simulink model "bldc_sim_2024a_v1"  (R2024b)
settings: Solver=VariableStepAuto  StartTime=0.0  StopTime=0.5  FixedStep=1e-6  MaxStep=1e-4  RelTol=1e-3
values from neighbouring files (symbols this model uses):
  D_m = 1e-5    (= 1e-05)    [setup_motor_params.m]
  J = 12e-4    (= 0.0012)    [setup_motor_params.m]
  L_ss = 0.45e-3    (= 0.00045)    [setup_motor_params.m]
  lambda_m = 21.5e-3    (= 0.0215)    [setup_motor_params.m]
  P = 8    [setup_motor_params.m]
  phi_A_deg = 9.0 * 0    (= 0)    [setup_motor_params.m]
  phi_B_deg = -1.0 * 0    (= 0)    [setup_motor_params.m]
  phi_C_deg = 7.0* 0    (= 0)    [setup_motor_params.m]
  R_s = 0.15    [setup_motor_params.m]
  tau_s = L_ss/R_s    (= 0.003)    [setup_motor_params.m]
  Ts_motor = 1e-6    (= 1e-06)    [setup_motor_params.m]
libraries: nesl_utility x13, fl_lib x10, ee_lib x8, spsPWMGeneratorDCDCLib x2
settings Model: Creator=Aether  LastModifiedBy=Aether

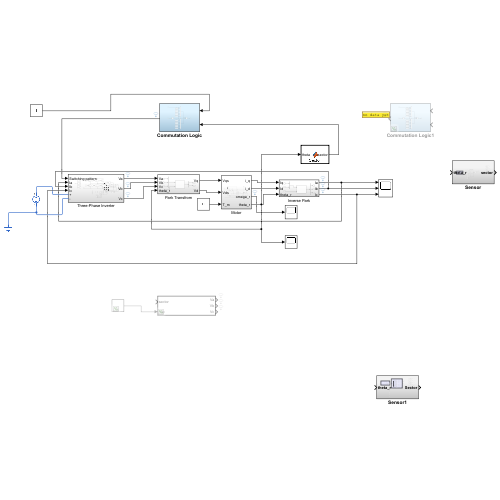
[thumbnail: Simulink's stored preview of the top-level diagram]
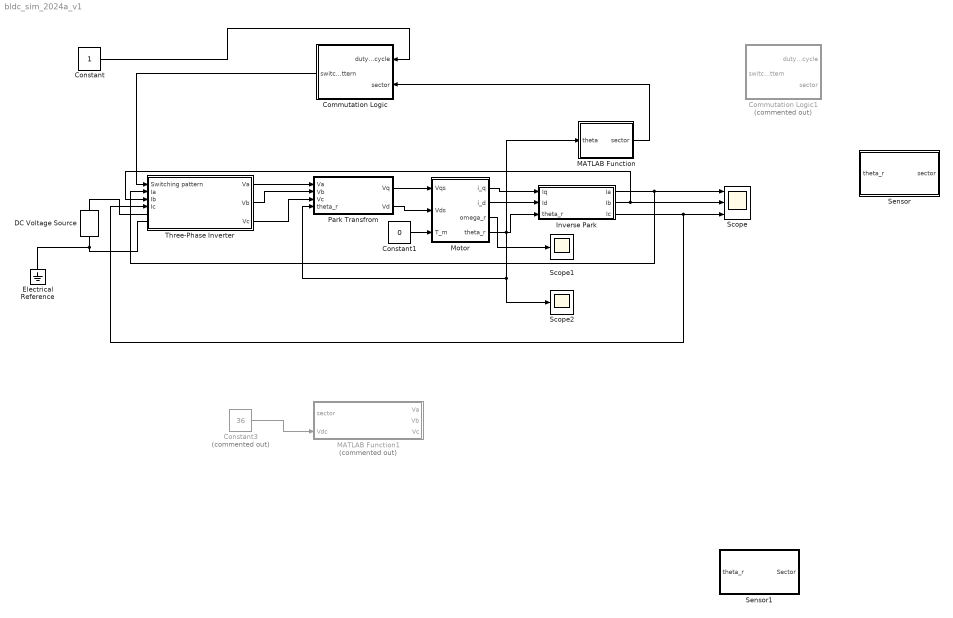
== system bldc_sim_2024a_v1 ==
  Commutation Logic : Subsystem
  Commutation Logic1 : Subsystem  Commented=on
  Constant : Constant
  Constant1 : Constant  Value=0
  Constant3 : Constant  Commented=on  Value=36
  DC Voltage Source : ee_lib/Additional Components/SPICE Sources/DC Voltage Source  DC=36 V
  Electrical Reference : fl_lib/Electrical/Electrical Elements/Electrical Reference
  Inverse Park : Subsystem
  MATLAB Function : MATLAB Function  TreatAsAtomicUnit=on
  MATLAB Function1 : MATLAB Function  Commented=on  TreatAsAtomicUnit=on
  Motor : Subsystem
  Park Transfrom : Subsystem
  Scope : Scope  NumInputPorts=3
  Scope1 : Scope
  Scope2 : Scope
  Sensor : Subsystem
  Sensor1 : Subsystem
  Three-Phase Inverter : Subsystem
  wires:
  Park Transfrom/1(Vq) -> Motor/1(Vqs)
  Park Transfrom/2(Vd) -> Motor/2(Vds)
  Motor/1(i_q) -> Inverse Park/1(Iq)
  Motor/2(i_d) -> Inverse Park/2(Id)
  Motor/4(theta_r) -> MATLAB Function/1(theta), Scope2/1, Park Transfrom/4(theta_r), Inverse Park/3(theta_r)
  Inverse Park/1(Ia) -> Three-Phase Inverter/2(Ia), Scope/1
  Inverse Park/2(Ib) -> Scope/2, Three-Phase Inverter/3(Ib)
  Inverse Park/3(Ic) -> Three-Phase Inverter/4(Ic), Scope/3
  Constant1/1 -> Motor/3(T_m)
  Motor/3(omega_r) -> Scope1/1
  Constant3/1 -> MATLAB Function1/2(Vdc)
  Three-Phase Inverter/1(Va) -> Park Transfrom/1(Va)
  Three-Phase Inverter/2(Vb) -> Park Transfrom/2(Vb)
  Three-Phase Inverter/3(Vc) -> Park Transfrom/3(Vc)
  Constant/1 -> Commutation Logic/1(duty_cycle)
  MATLAB Function/1(sector) -> Commutation Logic/2(sector)
  Commutation Logic/1("  switching_pattern") -> Three-Phase Inverter/1(Switching pattern)
  connections:
  DC Voltage Source/LConn1 -- Three-Phase Inverter/LConn1
  DC Voltage Source/RConn1 -- Electrical Reference/LConn1 -- Three-Phase Inverter/LConn2

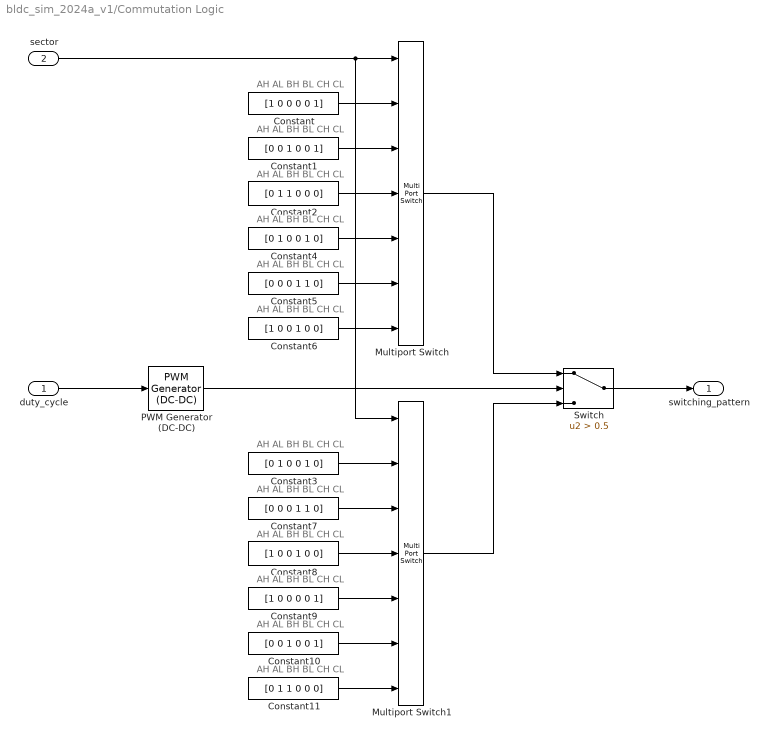
== system bldc_sim_2024a_v1/Commutation Logic ==
  note: AH AL BH BL CH CL
  note: AH AL BH BL CH CL
  note: AH AL BH BL CH CL
  note: AH AL BH BL CH CL
  note: AH AL BH BL CH CL
  note: AH AL BH BL CH CL
  note: AH AL BH BL CH CL
  note: AH AL BH BL CH CL
  note: AH AL BH BL CH CL
  note: AH AL BH BL CH CL
  note: AH AL BH BL CH CL
  note: AH AL BH BL CH CL
  duty_cycle : Inport
  sector : Inport  Port=2
  Constant : Constant  Value=[1 0 0 0 0 1]
  Constant1 : Constant  Value=[0 0 1 0 0 1]
  Constant10 : Constant  Value=[0 0 1 0 0 1]
  Constant11 : Constant  Value=[0 1 1 0 0 0]
  Constant2 : Constant  Value=[0 1 1 0 0 0]
  Constant3 : Constant  Value=[0 1 0 0 1 0]
  Constant4 : Constant  Value=[0 1 0 0 1 0]
  Constant5 : Constant  Value=[0 0 0 1 1 0]
  Constant6 : Constant  Value=[1 0 0 1 0 0]
  Constant7 : Constant  Value=[0 0 0 1 1 0]
  Constant8 : Constant  Value=[1 0 0 1 0 0]
  Constant9 : Constant  Value=[1 0 0 0 0 1]
  Multiport Switch : MultiPortSwitch  Inputs=6  SaturateOnIntegerOverflow=off  InputSameDT=off
  Multiport Switch1 : MultiPortSwitch  Inputs=6  SaturateOnIntegerOverflow=off  InputSameDT=off
  PWM Generator (DC-DC) : spsPWMGeneratorDCDCLib/PWM Generator (DC-DC)  Fsw=1e4  Ts=Ts_motor
  Switch : Switch  Criteria=u2 > Threshold  Threshold=0.5  SaturateOnIntegerOverflow=off  InputSameDT=off
  "  switching_pattern" : Outport  VectorParamsAs1DForOutWhenUnconnected=off
  wires:
  Constant6/1 -> Multiport Switch/7
  Constant4/1 -> Multiport Switch/5
  sector/1 -> Multiport Switch1/1, Multiport Switch/1
  Constant1/1 -> Multiport Switch/3
  Constant2/1 -> Multiport Switch/4
  Constant5/1 -> Multiport Switch/6
  Constant/1 -> Multiport Switch/2
  Constant9/1 -> Multiport Switch1/5
  Constant11/1 -> Multiport Switch1/7
  Constant3/1 -> Multiport Switch1/2
  Constant7/1 -> Multiport Switch1/3
  Constant10/1 -> Multiport Switch1/6
  Constant8/1 -> Multiport Switch1/4
  PWM Generator (DC-DC)/1 -> Switch/2
  Switch/1 -> "  switching_pattern"/1
  Multiport Switch/1 -> Switch/1
  Multiport Switch1/1 -> Switch/3
  duty_cycle/1 -> PWM Generator (DC-DC)/1

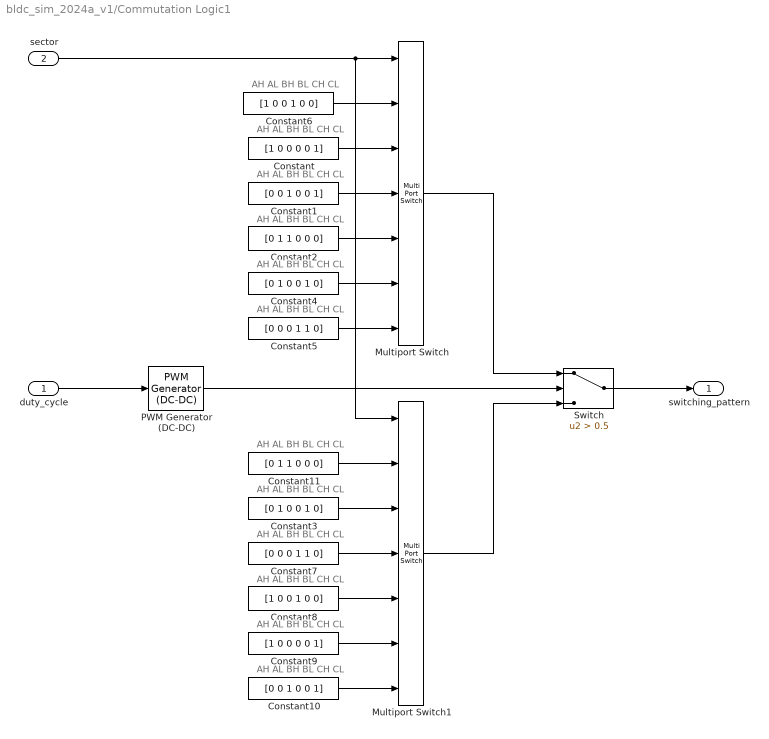
== system bldc_sim_2024a_v1/Commutation Logic1 ==
  note: AH AL BH BL CH CL
  note: AH AL BH BL CH CL
  note: AH AL BH BL CH CL
  note: AH AL BH BL CH CL
  note: AH AL BH BL CH CL
  note: AH AL BH BL CH CL
  note: AH AL BH BL CH CL
  note: AH AL BH BL CH CL
  note: AH AL BH BL CH CL
  note: AH AL BH BL CH CL
  note: AH AL BH BL CH CL
  note: AH AL BH BL CH CL
  duty_cycle : Inport
  sector : Inport  Port=2
  Constant : Constant  Value=[1 0 0 0 0 1]
  Constant1 : Constant  Value=[0 0 1 0 0 1]
  Constant10 : Constant  Value=[0 0 1 0 0 1]
  Constant11 : Constant  Value=[0 1 1 0 0 0]
  Constant2 : Constant  Value=[0 1 1 0 0 0]
  Constant3 : Constant  Value=[0 1 0 0 1 0]
  Constant4 : Constant  Value=[0 1 0 0 1 0]
  Constant5 : Constant  Value=[0 0 0 1 1 0]
  Constant6 : Constant  Value=[1 0 0 1 0 0]
  Constant7 : Constant  Value=[0 0 0 1 1 0]
  Constant8 : Constant  Value=[1 0 0 1 0 0]
  Constant9 : Constant  Value=[1 0 0 0 0 1]
  Multiport Switch : MultiPortSwitch  Inputs=6  SaturateOnIntegerOverflow=off  InputSameDT=off
  Multiport Switch1 : MultiPortSwitch  Inputs=6  SaturateOnIntegerOverflow=off  InputSameDT=off
  PWM Generator (DC-DC) : spsPWMGeneratorDCDCLib/PWM Generator (DC-DC)  Fsw=1e4  Ts=Ts_motor
  Switch : Switch  Criteria=u2 > Threshold  Threshold=0.5  SaturateOnIntegerOverflow=off  InputSameDT=off
  "  switching_pattern" : Outport  VectorParamsAs1DForOutWhenUnconnected=off
  wires:
  sector/1 -> Multiport Switch1/1, Multiport Switch/1
  PWM Generator (DC-DC)/1 -> Switch/2
  Switch/1 -> "  switching_pattern"/1
  Multiport Switch/1 -> Switch/1
  Multiport Switch1/1 -> Switch/3
  duty_cycle/1 -> PWM Generator (DC-DC)/1
  Constant5/1 -> Multiport Switch/7
  Constant4/1 -> Multiport Switch/6
  Constant2/1 -> Multiport Switch/5
  Constant1/1 -> Multiport Switch/4
  Constant/1 -> Multiport Switch/3
  Constant6/1 -> Multiport Switch/2
  Constant10/1 -> Multiport Switch1/7
  Constant9/1 -> Multiport Switch1/6
  Constant8/1 -> Multiport Switch1/5
  Constant7/1 -> Multiport Switch1/4
  Constant3/1 -> Multiport Switch1/3
  Constant11/1 -> Multiport Switch1/2

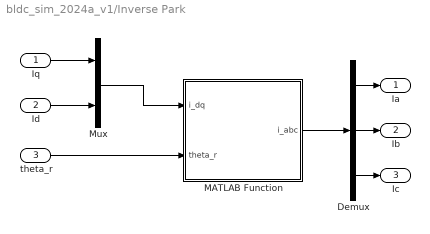
== system bldc_sim_2024a_v1/Inverse Park ==
  Iq : Inport
  Id : Inport  Port=2
  theta_r : Inport  Port=3
  Demux : Demux  Outputs=3
  MATLAB Function : MATLAB Function  TreatAsAtomicUnit=on
  Mux : Mux  Inputs=2
  Ia : Outport
  Ib : Outport  Port=2
  Ic : Outport  Port=3
  wires:
  Mux/1 -> MATLAB Function/1(i_dq)
  theta_r/1 -> MATLAB Function/2(theta_r)
  MATLAB Function/1(i_abc) -> Demux/1
  Id/1 -> Mux/2
  Iq/1 -> Mux/1
  Demux/1 -> Ia/1
  Demux/2 -> Ib/1
  Demux/3 -> Ic/1

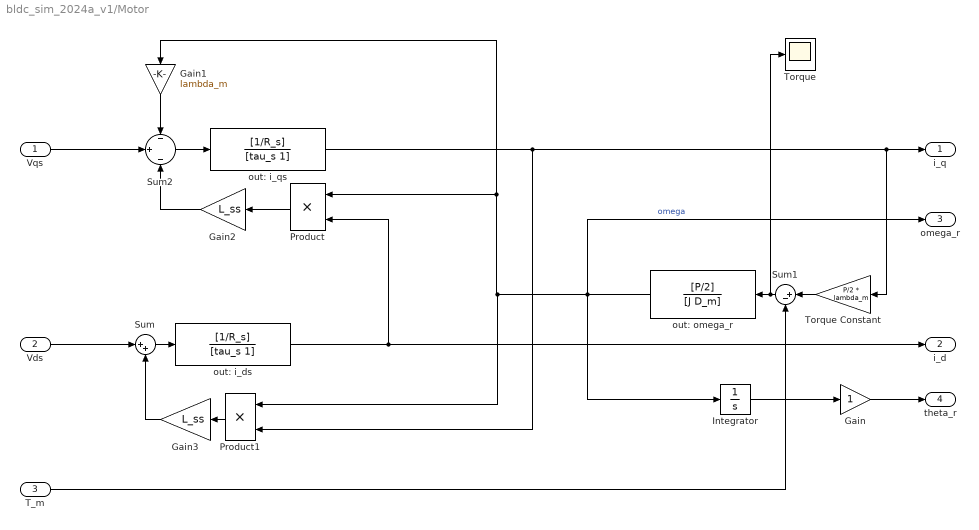
== system bldc_sim_2024a_v1/Motor ==
  Vqs : Inport
  Vds : Inport  Port=2
  T_m : Inport  Port=3
  Gain : Gain
  Gain1 : Gain  Gain=lambda_m
  Gain2 : Gain  Gain=L_ss
  Gain3 : Gain  Gain=L_ss
  Integrator : Integrator
  Product : Product
  Product1 : Product
  Sum : Sum  Inputs=|++
  Sum1 : Sum  Inputs=|+-
  Sum2 : Sum  Inputs=-|+|-
  Torque : Scope
  Torque Constant : Gain  Gain=P/2 * lambda_m
  out: i_ds : TransferFcn  Numerator=[1/R_s]  Denominator=[tau_s 1]
  out: i_qs : TransferFcn  Numerator=[1/R_s]  Denominator=[tau_s 1]
  out: omega_r : TransferFcn  Numerator=[P/2]  Denominator=[J D_m]
  i_q : Outport
  i_d : Outport  Port=2
  omega_r : Outport  Port=3
  theta_r : Outport  Port=4
  wires:
  Sum2/1 -> out: i_qs/1
  Vqs/1 -> Sum2/2
  out: omega_r/1 -> omega_r/1, Integrator/1, Product1/1, Product/1, Gain1/1  "omega"
  Gain1/1 -> Sum2/1
  out: i_ds/1 -> Product/2, i_d/1
  Integrator/1 -> Gain/1
  T_m/1 -> Sum1/2
  Sum1/1 -> Torque/1, out: omega_r/1
  Sum/1 -> out: i_ds/1
  Torque Constant/1 -> Sum1/1
  Product/1 -> Gain2/1
  out: i_qs/1 -> Product1/2, i_q/1, Torque Constant/1
  Vds/1 -> Sum/1
  Gain/1 -> theta_r/1
  Product1/1 -> Gain3/1
  Gain3/1 -> Sum/2
  Gain2/1 -> Sum2/3

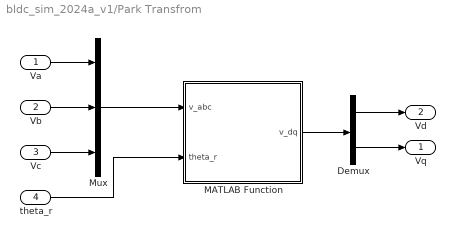
== system bldc_sim_2024a_v1/Park Transfrom ==
  Va : Inport
  Vb : Inport  Port=2
  Vc : Inport  Port=3
  theta_r : Inport  Port=4
  Demux : Demux  Outputs=2
  MATLAB Function : MATLAB Function  TreatAsAtomicUnit=on
  Mux : Mux  Inputs=3
  Vq : Outport
  Vd : Outport  Port=2
  wires:
  theta_r/1 -> MATLAB Function/2(theta_r)
  Vb/1 -> Mux/2
  Va/1 -> Mux/1
  Vc/1 -> Mux/3
  Mux/1 -> MATLAB Function/1(v_abc)
  MATLAB Function/1(v_dq) -> Demux/1
  Demux/1 -> Vd/1
  Demux/2 -> Vq/1

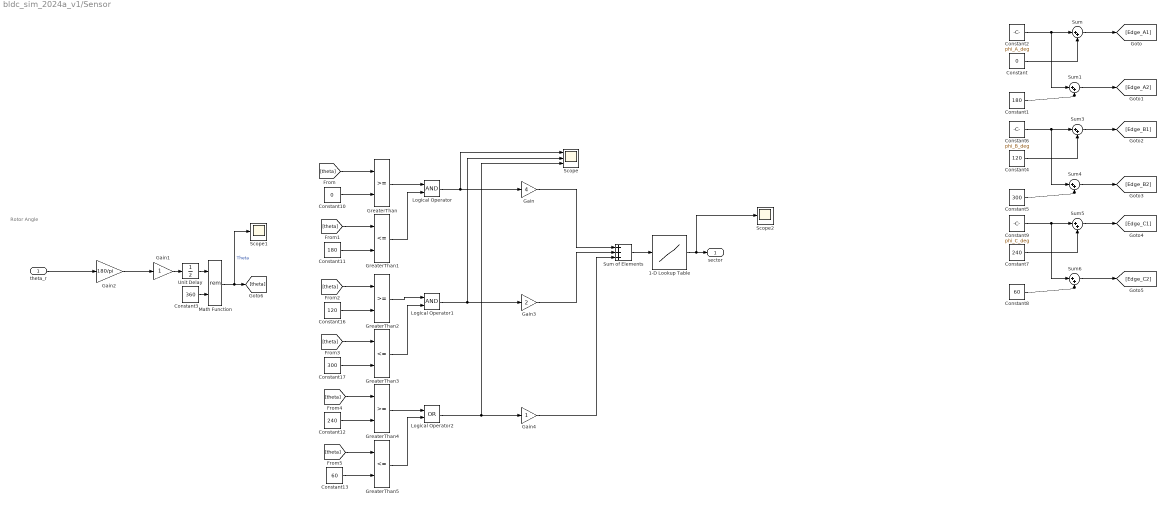
== system bldc_sim_2024a_v1/Sensor ==
  note: Rotor Angle
  theta_r : Inport
  1-D Lookup Table : Lookup_n-D  NumberOfTableDimensions=1  BreakpointsForDimension1=[1 2 3 4 5 6]  Table=[6 4 5 2 1 3]  ExtrapMethod=Clip  InternalRulePriority=Speed  RndMeth=Simplest
  Constant : Constant  Value=0
  Constant1 : Constant  Value=180
  Constant10 : Constant  Value=0
  Constant11 : Constant  Value=180
  Constant12 : Constant  Value=240
  Constant13 : Constant  Value=60
  Constant16 : Constant  Value=120
  Constant17 : Constant  Value=300
  Constant2 : Constant  Value=phi_A_deg
  Constant3 : Constant  Value=360
  Constant4 : Constant  Value=120
  Constant5 : Constant  Value=300
  Constant6 : Constant  Value=phi_B_deg
  Constant7 : Constant  Value=240
  Constant8 : Constant  Value=60
  Constant9 : Constant  Value=phi_C_deg
  Gain : Gain  Gain=4
  Gain1 : Gain
  Gain2 : Gain  Gain=180/pi
  Gain3 : Gain  Gain=2
  Gain4 : Gain
  GreaterThan : RelationalOperator  OutDataTypeStr=boolean  RndMeth=Simplest  InputSameDT=off
  GreaterThan1 : RelationalOperator  Operator=<=  OutDataTypeStr=boolean  RndMeth=Simplest  InputSameDT=off
  GreaterThan2 : RelationalOperator  OutDataTypeStr=boolean  RndMeth=Simplest  InputSameDT=off
  GreaterThan3 : RelationalOperator  Operator=<=  OutDataTypeStr=boolean  RndMeth=Simplest  InputSameDT=off
  GreaterThan4 : RelationalOperator  OutDataTypeStr=boolean  RndMeth=Simplest  InputSameDT=off
  GreaterThan5 : RelationalOperator  Operator=<=  OutDataTypeStr=boolean  RndMeth=Simplest  InputSameDT=off
  Logical Operator : Logic  AllPortsSameDT=off  OutDataTypeStr=boolean
  Logical Operator1 : Logic  AllPortsSameDT=off  OutDataTypeStr=boolean
  Logical Operator2 : Logic  Operator=OR  AllPortsSameDT=off  OutDataTypeStr=boolean
  Math Function : Math  Operator=rem  SignedPower=on
  Scope : Scope  NumInputPorts=3
  Scope1 : Scope
  Scope2 : Scope
  Sum{,1,3..6} (6 alike) : Sum  Inputs=|++
  Sum of Elements : Sum  Inputs=+++
  Unit Delay : UnitDelay  SampleTime=Ts_motor  HasFrameUpgradeWarning=on
  sector : Outport
  wires:
  Gain2/1 -> Gain1/1
  Constant3/1 -> Math Function/2
  Gain1/1 -> Unit Delay/1
  Unit Delay/1 -> Math Function/1
  Constant/1 -> Sum/2
  Constant2/1 -> Sum1/1, Sum/1
  Constant1/1 -> Sum1/2
  Sum/1 -> [Edge_A1]
  Sum1/1 -> [Edge_A2]
  Constant6/1 -> Sum4/1, Sum3/1
  Constant5/1 -> Sum4/2
  Constant4/1 -> Sum3/2
  Sum3/1 -> [Edge_B1]
  Sum4/1 -> [Edge_B2]
  Constant9/1 -> Sum6/1, Sum5/1
  Constant8/1 -> Sum6/2
  Constant7/1 -> Sum5/2
  Sum5/1 -> [Edge_C1]
  Sum6/1 -> [Edge_C2]
  theta_r/1 -> Gain2/1
  Math Function/1 -> Scope1/1, [theta]  "Theta"
  GreaterThan/1 -> Logical Operator/1
  [theta] -> GreaterThan/1
  Constant11/1 -> GreaterThan1/2
  GreaterThan1/1 -> Logical Operator/2
  GreaterThan3/1 -> Logical Operator1/2
  GreaterThan2/1 -> Logical Operator1/1
  GreaterThan4/1 -> Logical Operator2/1
  GreaterThan5/1 -> Logical Operator2/2
  Logical Operator/1 -> Scope/1, Gain/1
  Logical Operator1/1 -> Scope/2, Gain3/1
  Logical Operator2/1 -> Scope/3, Gain4/1
  Sum of Elements/1 -> 1-D Lookup Table/1
  Gain/1 -> Sum of Elements/1
  Gain3/1 -> Sum of Elements/2
  Gain4/1 -> Sum of Elements/3
  1-D Lookup Table/1 -> Scope2/1, sector/1
  Constant10/1 -> GreaterThan/2
  [theta] -> GreaterThan1/1
  [theta] -> GreaterThan2/1
  Constant16/1 -> GreaterThan2/2
  [theta] -> GreaterThan3/1
  Constant17/1 -> GreaterThan3/2
  [theta] -> GreaterThan4/1
  Constant12/1 -> GreaterThan4/2
  [theta] -> GreaterThan5/1
  Constant13/1 -> GreaterThan5/2

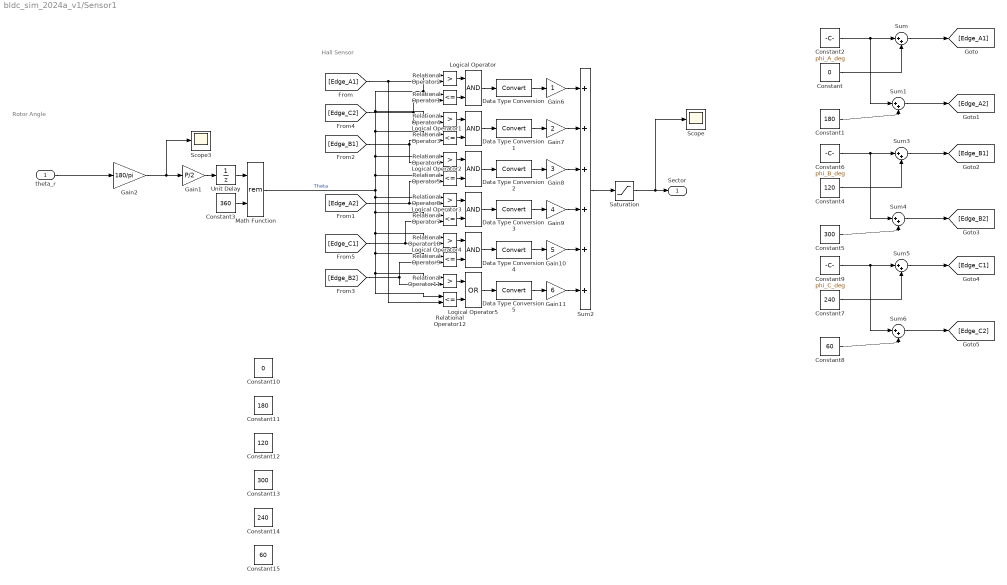
== system bldc_sim_2024a_v1/Sensor1 ==
  note: Rotor Angle
  note: Hall Sensor
  theta_r : Inport
  Constant : Constant  Value=0
  Constant1 : Constant  Value=180
  Constant10 : Constant  Value=0
  Constant11 : Constant  Value=180
  Constant12 : Constant  Value=120
  Constant13 : Constant  Value=300
  Constant14 : Constant  Value=240
  Constant15 : Constant  Value=60
  Constant2 : Constant  Value=phi_A_deg
  Constant3 : Constant  Value=360
  Constant4 : Constant  Value=120
  Constant5 : Constant  Value=300
  Constant6 : Constant  Value=phi_B_deg
  Constant7 : Constant  Value=240
  Constant8 : Constant  Value=60
  Constant9 : Constant  Value=phi_C_deg
  Data Type Conversion{,1..5} (6 alike) : DataTypeConversion
  Gain1 : Gain  Gain=P/2
  Gain10 : Gain  Gain=5  SaturateOnIntegerOverflow=on  OutDataTypeStr=Inherit: Same as input  ParamDataTypeStr=Inherit: Same as input
  Gain11 : Gain  Gain=6  SaturateOnIntegerOverflow=on  OutDataTypeStr=Inherit: Same as input  ParamDataTypeStr=Inherit: Same as input
  Gain2 : Gain  Gain=180/pi
  Gain6 : Gain  SaturateOnIntegerOverflow=on  OutDataTypeStr=Inherit: Same as input  ParamDataTypeStr=Inherit: Same as input
  Gain7 : Gain  Gain=2  SaturateOnIntegerOverflow=on  OutDataTypeStr=Inherit: Same as input  ParamDataTypeStr=Inherit: Same as input
  Gain8 : Gain  Gain=3  SaturateOnIntegerOverflow=on  OutDataTypeStr=Inherit: Same as input  ParamDataTypeStr=Inherit: Same as input
  Gain9 : Gain  Gain=4  SaturateOnIntegerOverflow=on  OutDataTypeStr=Inherit: Same as input  ParamDataTypeStr=Inherit: Same as input
  Logical Operator{,1..4} (5 alike) : Logic
  Logical Operator5 : Logic  Operator=OR
  Math Function : Math  Operator=rem  SignedPower=on
  Relational Operator{1,3,5,7,9,12} (6 alike) : RelationalOperator  Operator=<=
  Relational Operator{2,4,6,8,10..11} (6 alike) : RelationalOperator  Operator=>
  Saturation : Saturate  UpperLimit=6  LowerLimit=1
  Scope : Scope
  Scope3 : Scope
  Sum{,1,3..6} (6 alike) : Sum  Inputs=|++
  Sum2 : Sum  Inputs=++++++  InputSameDT=on  SaturateOnIntegerOverflow=on  OutDataTypeStr=Inherit: Same as first input
  Unit Delay : UnitDelay  SampleTime=Ts_motor  HasFrameUpgradeWarning=on
  Sector : Outport
  wires:
  Saturation/1 -> Scope/1, Sector/1
  Math Function/1 -> Relational Operator2/1, Relational Operator1/1, Relational Operator4/1, Relational Operator3/1, Relational Operator6/1, Relational Operator5/1, Relational Operator12/1, Relational Operator11/1, Relational Operator9/1, Relational Operator10/1, Relational Operator7/1, Relational Operator8/1  "Theta"
  Data Type Conversion5/1 -> Gain11/1
  Data Type Conversion4/1 -> Gain10/1
  Data Type Conversion3/1 -> Gain9/1
  Data Type Conversion2/1 -> Gain8/1
  Data Type Conversion1/1 -> Gain7/1
  Data Type Conversion/1 -> Gain6/1
  Relational Operator2/1 -> Logical Operator/1
  Relational Operator1/1 -> Logical Operator/2
  Logical Operator/1 -> Data Type Conversion/1
  [Edge_A1] -> Relational Operator12/2, Relational Operator2/2
  Relational Operator4/1 -> Logical Operator1/1
  Relational Operator3/1 -> Logical Operator1/2
  Logical Operator1/1 -> Data Type Conversion1/1
  [Edge_C2] -> Relational Operator1/2, Relational Operator4/2
  Relational Operator6/1 -> Logical Operator2/1
  Relational Operator5/1 -> Logical Operator2/2
  Logical Operator2/1 -> Data Type Conversion2/1
  Relational Operator8/1 -> Logical Operator3/1
  Relational Operator7/1 -> Logical Operator3/2
  Logical Operator3/1 -> Data Type Conversion3/1
  Relational Operator10/1 -> Logical Operator4/1
  Relational Operator9/1 -> Logical Operator4/2
  Logical Operator4/1 -> Data Type Conversion4/1
  Relational Operator11/1 -> Logical Operator5/1
  Relational Operator12/1 -> Logical Operator5/2
  Logical Operator5/1 -> Data Type Conversion5/1
  Gain6/1 -> Sum2/1
  Gain7/1 -> Sum2/2
  Gain8/1 -> Sum2/3
  Gain9/1 -> Sum2/4
  Gain10/1 -> Sum2/5
  Gain11/1 -> Sum2/6
  Sum2/1 -> Saturation/1
  Gain2/1 -> Scope3/1, Gain1/1
  Constant3/1 -> Math Function/2
  Gain1/1 -> Unit Delay/1
  Unit Delay/1 -> Math Function/1
  Constant/1 -> Sum/2
  Constant2/1 -> Sum1/1, Sum/1
  Constant1/1 -> Sum1/2
  Sum/1 -> [Edge_A1]
  Sum1/1 -> [Edge_A2]
  Constant6/1 -> Sum4/1, Sum3/1
  Constant5/1 -> Sum4/2
  Constant4/1 -> Sum3/2
  Sum3/1 -> [Edge_B1]
  Sum4/1 -> [Edge_B2]
  Constant9/1 -> Sum6/1, Sum5/1
  Constant8/1 -> Sum6/2
  Constant7/1 -> Sum5/2
  Sum5/1 -> [Edge_C1]
  Sum6/1 -> [Edge_C2]
  [Edge_B1] -> Relational Operator3/2, Relational Operator6/2
  [Edge_A2] -> Relational Operator5/2, Relational Operator8/2
  [Edge_C1] -> Relational Operator7/2, Relational Operator10/2
  [Edge_B2] -> Relational Operator11/2, Relational Operator9/2
  theta_r/1 -> Gain2/1

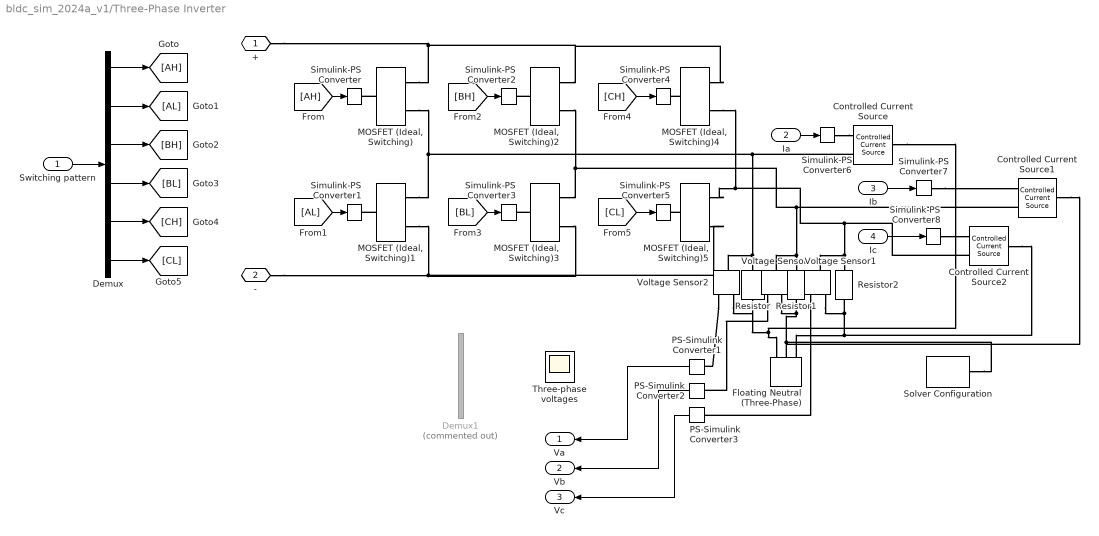
== system bldc_sim_2024a_v1/Three-Phase Inverter ==
  Switching pattern : Inport
  Ia : Inport  Port=2
  Ib : Inport  Port=3
  Ic : Inport  Port=4
  Controlled Current Source : fl_lib/Electrical/Electrical Sources/Controlled Current Source
  Controlled Current Source1 : fl_lib/Electrical/Electrical Sources/Controlled Current Source
  Controlled Current Source2 : fl_lib/Electrical/Electrical Sources/Controlled Current Source
  Demux : Demux  Outputs=6
  Demux1 : Demux  Commented=on  Outputs=3
  Floating Neutral (Three-Phase) : ee_lib/Connectors & References/Floating Neutral (Three-Phase)  G_parasitic=1e-12 1/Ohm
      settings: InternalSimscapePortConfiguration="{\"Bottom\":[],\"Left\":[{\"id\":\"a\",\"label\":\"a\",\"type\":\"foundation.electrical.electrical\"},{\"id\":\"b\",\"label\":\"b\",\"type\":\"foundation.electrical.electrical\"},{\"id\":\"c\",\"label\":\"c\",\"type\":\"foundation.electrical.electrical\"}],\"Right\":[],\"Top\":[]}"
  MOSFET (Ideal, Switching){,1..5} (6 alike) : ee_lib/Semiconductors & Converters/MOSFET (Ideal, Switching)  port_option=ee.enum.controlport.ps  Rds=0.01 Ohm  Goff=1e-6 1/Ohm  Vth=0.5 V  diode_param=ee.enum.semiconductors.protectionDiode.nodynamics  diode_Vf=0.1 V  diode_Ron=0.001 Ohm  diode_Goff=1e-5 1/Ohm  diode_C=50e-9 F  diode_iRM=-235 A  diode_iF=300 A  diode_idot=-50 A/us  diode_trr_param=ee.enum.converters.diodeReverseParam.trr_factor  diode_trr_factor=3  diode_trr=15 us  diode_Qrr=1500 s*uA  ids_specify=off  ids_priority=None  ids=0 A  ids_nominal_specify=off  ids_nominal_value=1  ids_nominal_unit=A  vds_specify=off  vds_priority=None  vds=0 V  vds_nominal_specify=off  vds_nominal_value=1  vds_nominal_unit=V  vgs_specify=off  vgs_priority=None  vgs=0 V  vgs_nominal_specify=off  vgs_nominal_value=1  vgs_nominal_unit=V  thermal_loss_option=ee.enum.converters.thermalLossOption.constantvalues  Von_data=[0, 1.8, 3.2, 6, 10, 16; 0, 2, 5.5, 9.5, 15, 25] V  Tj=[298.15, 448.15] K  Iout_data=[0, 20, 40, 60, 80, 100] A  Eon_data=[0, 55.04, 124.57, 235.53, 362.12; 0, 71.25, 161.25, 304.88, 468.75] * 1e-6 J  Eoff_data=[0, 18, 30, 56.1, 76.5; 0, 22.5, 37.5, 70.13, 95.63] * 1e-6 J  Eon_data_3D=[zeros(2, 5, 3)] J  Eoff_data_3D=[zeros(2, 5, 3)] J  Tj_loss=[298.15, 448.15] K  Iout_data_loss=[0, 10, 20, 30, 40] A  tabulateWithVds=false  Vds_loss=[0, 150, 300] V  Eon_scalar=22.86e-3 J  Eoff_scalar=17.14e-3 J  Voff=300 V  Iout_scalar=600 A  useCurrentFromPreviousCycle=false  useVoltageFromPreviousCycle=false  diodeModelType=ee.enum.converters.diodeModelType.pwl  diodeTableType=ee.enum.diode.tableType.IfMat  diode_ReverseIVType=ee.enum.diode.diodeReverseIV.constant  diode_IfMat=[.07, .12, .19, 1.75, 4.24, 7.32, 11.2; .16, .3, .72, 2.14, 4.02, 6.35, 9.12] A  diode_VfMat=[.9, 1.15, 1.25, 1.5, 1.75, 2.17, 2.6, 2.85; .58, .68, .75, 1.1, 1.38, 1.77, 2.27, 2.7] V  diode_TjVec=[25, 125] degC  diode_VfVec=[.5, .7, .9, 1.3, 1.7, 2.1, 2.5] V  diode_IfVec=[.1, .2, .5, 1, 2, 4, 7, 10] A  diode_IrMat=[1e-06, 2e-06, 5e-06, 1e-05, 2.5e-05, 5e-05, .0001; 2e-06, 5e-06, 1e-05, 4e-05, 8e-05, .0002, .0005] A  diode_VrMat=[10, 100, 200, 250, 300, 325, 350; 10, 70, 160, 220, 270, 300, 320] V  diode_VrVec=[10, 20, 40, 50, 70, 80, 100] V  diode_IrVec=[1e-06, 2e-06, 5e-06, 1e-05, 2e-05, 5e-05, .0001] A  diode_Vr=-600 V  diode_Ls=150 nH  diode_Erec=0.03 J  diode_rec_loss_model=ee.enum.diode.reverseRecoveryModel.fixed  diode_ErecVal=0 J  diode_scaleWithIandV=true  diode_ErecMat=zeros(2, 3) J  diode_TjrecVec=[298.15, 398.15] K  diode_IfrecVec=[.1, 1, 10] A  diode_IrecVal=10 A  diode_VrecVal=10 V  diode_tFilter=1 / 1000 / 100 s  separateThermalPortForDiode=false  thermal_network_parameterization=ee.enum.thermalNetworkTopology.external  Rth=[.03, .2] K/W  Rth_Cauer=[.03, .1, .2] K/W  Rth_Foster=[.03, .2] K/W  thermal_mass_parameterization=ee.enum.thermalNetwork.timeconstant  thermal_mass=[3, 25] J/K  thermal_mass_Cauer=[3, 10, 25] J/K  thermal_mass_Foster=[33, 50] J/K  thermal_time_constant=[.1, 5] s  thermal_time_constant_Cauer=[.1, 1, 5] s  thermal_time_constant_Foster=[1, 10] s  thermal_mass_initial_temperatures=[25, 25] degC  thermal_mass_initial_temperatures_Cauer=[25, 25, 25] degC  junction_thermal_mass=0.1 J/K  Tvec_initial_Foster=[25, 25, 25, 25] degC  RthDiode=[.03, .2] K/W  RthCauerDiode=[.03, .1, .2] K/W  RthFosterDiode=[.03, .2] K/W  thermalMassDiode=[3, 25] J/K  thermalMassCauerDiode=[3, 10, 25] J/K  thermalMassFosterDiode=[33, 50] J/K  thermalTauDiode=[.1, 5] s  thermalTauCauerDiode=[.1, 1, 5] s  thermalTauFosterDiode=[1, 10] s  thermalMassInitTempDiode=[25, 25] degC  thermalMassInitTempCauerDiode=[25, 25, 25] degC  junctionthermalMassDiode=0.1 J/K  TVecInitialFosterDiode=[25, 25, 25, 25] degC  no_thermal_network=0  mosfet_junction_temperature_specify=off  mosfet_junction_temperature_priority=None  mosfet_junction_temperature=25 degC  mosfet_junction_temperature_nominal_specify=off  mosfet_junction_temperature_nominal_value=1  mosfet_junction_temperature_nominal_unit=degC  diode_junction_temperature_specify=off  diode_junction_temperature_priority=None  diode_junction_temperature=25 degC  diode_junction_temperature_nominal_specify=off  diode_junction_temperature_nominal_value=1  diode_junction_temperature_nominal_unit=degC  Qj_specify=off  Qj_priority=None  Qj=0 W  Qj_nominal_specify=off  Qj_nominal_value=1  Qj_nominal_unit=W  accumulatedSwitchingLosses_specify=off  accumulatedSwitchingLosses_priority=None  accumulatedSwitchingLosses=0 J
  PS-Simulink Converter1 : nesl_utility/PS-Simulink Converter  PhysicalDomain=network_engine_domain  SubClassName=ps_output  LeftPortType=input  RightPortType=output  PseudoPeriodic=off  Frequencies=[]  VectorFormat=1-D array  Unit=1  AffineConversion=off
  PS-Simulink Converter2 : nesl_utility/PS-Simulink Converter  PhysicalDomain=network_engine_domain  SubClassName=ps_output  LeftPortType=input  RightPortType=output  PseudoPeriodic=off  Frequencies=[]  VectorFormat=1-D array  Unit=1  AffineConversion=off
  PS-Simulink Converter3 : nesl_utility/PS-Simulink Converter  PhysicalDomain=network_engine_domain  SubClassName=ps_output  LeftPortType=input  RightPortType=output  PseudoPeriodic=off  Frequencies=[]  VectorFormat=1-D array  Unit=1  AffineConversion=off
  Resistor : fl_lib/Electrical/Electrical Elements/Resistor  R=1e5 Ohm  i_specify=off  i_priority=None  i=0 A  i_nominal_specify=off  i_nominal_value=1  i_nominal_unit=A  v_specify=off  v_priority=None  v=0 V  v_nominal_specify=off  v_nominal_value=1  v_nominal_unit=V
  Resistor1 : fl_lib/Electrical/Electrical Elements/Resistor  R=1e5 Ohm  i_specify=off  i_priority=None  i=0 A  i_nominal_specify=off  i_nominal_value=1  i_nominal_unit=A  v_specify=off  v_priority=None  v=0 V  v_nominal_specify=off  v_nominal_value=1  v_nominal_unit=V
  Resistor2 : fl_lib/Electrical/Electrical Elements/Resistor  R=1e5 Ohm  i_specify=off  i_priority=None  i=0 A  i_nominal_specify=off  i_nominal_value=1  i_nominal_unit=A  v_specify=off  v_priority=None  v=0 V  v_nominal_specify=off  v_nominal_value=1  v_nominal_unit=V
  Simulink-PS Converter{,1..8} (9 alike) : nesl_utility/Simulink-PS Converter  PhysicalDomain=network_engine_domain  SubClassName=ps_input  LeftPortType=input  RightPortType=output  PseudoPeriodic=off  Frequencies=[]  NoiseDistribution=none  NoiseParameters=[]  Unit=1  AffineConversion=off  FilteringAndDerivatives=provide  SimscapeFilterOrder=1  InputFilterTimeConstant=0.001  UdotUserProvided=0
  Solver Configuration : nesl_utility/Solver Configuration  PhysicalDomain=network_engine_domain  SubClassName=solver  LeftPortType=input  RightPortType=generic  Tones=[]  Harmonics=[]  SimulateNoise=off  Profile=off  UseLocalSampling=off  EnableSwitchedLinearOptims=on  FrequencyDomain=off  UseCCode=off  RelTol=0.001  AbsTol=0.001  MinStep=1e-09  ToWorkspace=off  RevertToSquareIcSolve=off  NumHomotopyIterations=100  PhasorMode=off  PhasorModeNumHarmonics=1  ConsistencySolver=NEWTON_XTOL_AFTER_FTOL  IndexReductionMethod=DerivativeReplacement  DoDC=off  ResidualTolerance=1e-09  ConsistencyTolSource=GLOBAL  ConsistencyAbsTol=0.001  ConsistencyRelTol=0.001  ConsistencyTolFactor=0.001  UseLocalSolver=off  LocalSolverChoice=NE_BACKWARD_EULER_ADVANCER  ResolveIndetEquations=on  FunctionEvalNumThread=1  LocalSolverSampleTime=0.001  DoFixedCost=off  MaxNonlinIter=3  MaxModeIter=2  ComputeImpulses=off  ImpulseIterations=2  LinearAlgebra=auto  LinearAlgebraNumThread=0  EquationFormulation=NE_TIME_EF  DelaysMemoryBudget=1024  AutomaticFiltering=on  FilteringTimeConstant=0.001  PartitionStorageMethod=AS_NEEDED  PartitionMemoryBudget=1024  PartitionMethod=ROBUST  MultibodyUseLocalSolver=off  MultibodyLocalSolverChoice=ODE1  MultibodyLocalSolverSampleTime=0.001
  Three-phase voltages : Scope
  Voltage Sensor : fl_lib/Electrical/Electrical Sensors/Voltage Sensor
  Voltage Sensor1 : fl_lib/Electrical/Electrical Sensors/Voltage Sensor
  Voltage Sensor2 : fl_lib/Electrical/Electrical Sensors/Voltage Sensor
  + : PMIOPort  Side=Left
  - : PMIOPort  Port=2  Side=Left
  Va : Outport
  Vb : Outport  Port=2
  Vc : Outport  Port=3
  wires:
  [BH] -> Simulink-PS Converter2/1
  [CL] -> Simulink-PS Converter5/1
  Switching pattern/1 -> Demux/1
  Demux/1 -> [AH]
  [AH] -> Simulink-PS Converter/1
  [AL] -> Simulink-PS Converter1/1
  Demux/5 -> [CH]
  Demux/4 -> [BL]
  [BL] -> Simulink-PS Converter3/1
  Demux/3 -> [BH]
  [CH] -> Simulink-PS Converter4/1
  Demux/2 -> [AL]
  Demux/6 -> [CL]
  PS-Simulink Converter1/1 -> Va/1
  PS-Simulink Converter2/1 -> Vb/1
  PS-Simulink Converter3/1 -> Vc/1
  Ia/1 -> Simulink-PS Converter6/1
  Ib/1 -> Simulink-PS Converter7/1
  Ic/1 -> Simulink-PS Converter8/1
  connections:
  "MOSFET (Ideal, Switching)4"/RConn1 -- "MOSFET (Ideal, Switching)2"/RConn1 -- "MOSFET (Ideal, Switching)"/RConn1 -- +/RConn1
  "MOSFET (Ideal, Switching)3"/LConn1 -- Simulink-PS Converter3/RConn1
  Controlled Current Source/RConn2 -- "MOSFET (Ideal, Switching)1"/RConn1 -- "MOSFET (Ideal, Switching)"/RConn2 -- Voltage Sensor2/LConn1 -- Resistor/LConn1
  "MOSFET (Ideal, Switching)5"/RConn2 -- "MOSFET (Ideal, Switching)3"/RConn2 -- "MOSFET (Ideal, Switching)1"/RConn2 -- -/RConn1
  Controlled Current Source1/RConn2 -- "MOSFET (Ideal, Switching)3"/RConn1 -- "MOSFET (Ideal, Switching)2"/RConn2 -- Voltage Sensor/LConn1 -- Resistor1/LConn1
  "MOSFET (Ideal, Switching)5"/LConn1 -- Simulink-PS Converter5/RConn1
  Controlled Current Source2/RConn2 -- "MOSFET (Ideal, Switching)5"/RConn1 -- "MOSFET (Ideal, Switching)4"/RConn2 -- Voltage Sensor1/LConn1 -- Resistor2/LConn1
  "MOSFET (Ideal, Switching)4"/LConn1 -- Simulink-PS Converter4/RConn1
  Voltage Sensor2/RConn1 -- PS-Simulink Converter1/LConn1
  "MOSFET (Ideal, Switching)"/LConn1 -- Simulink-PS Converter/RConn1
  "MOSFET (Ideal, Switching)1"/LConn1 -- Simulink-PS Converter1/RConn1
  "MOSFET (Ideal, Switching)2"/LConn1 -- Simulink-PS Converter2/RConn1
  Simulink-PS Converter6/RConn1 -- Controlled Current Source/RConn1
  Simulink-PS Converter7/RConn1 -- Controlled Current Source1/RConn1
  Simulink-PS Converter8/RConn1 -- Controlled Current Source2/RConn1
  Controlled Current Source/LConn1 -- Voltage Sensor2/RConn2 -- Resistor/RConn1 -- Floating Neutral (Three-Phase)/LConn1
  Floating Neutral (Three-Phase)/LConn2 -- Voltage Sensor/RConn2 -- Resistor1/RConn1 -- Solver Configuration/RConn1 -- Controlled Current Source1/LConn1
  Floating Neutral (Three-Phase)/LConn3 -- Controlled Current Source2/LConn1 -- Voltage Sensor1/RConn2 -- Resistor2/RConn1
  Voltage Sensor/RConn1 -- PS-Simulink Converter2/LConn1
  Voltage Sensor1/RConn1 -- PS-Simulink Converter3/LConn1

== matlab function bldc_sim_2024a_v1/Inverse Park/MATLAB Function ==
  data: i_dq input; i_abc output; theta_r input
function i_abc = inverse_park_transform(i_dq,theta_r)


th = theta_r;

K_inv = [ cos(th)                  sin(th);
          cos(th - 2*pi/3)         sin(th - 2*pi/3);
          cos(th + 2*pi/3)         sin(th + 2*pi/3) ];

i_abc = K_inv * i_dq;

end

== matlab function bldc_sim_2024a_v1/Park Transfrom/MATLAB Function ==
  data: v_abc input; v_dq output; theta_r input
function v_dq = park_transform(v_abc,theta_r)

th = theta_r;

K = (2/3) * [ cos(th)     cos(th - 2*pi/3)     cos(th + 2*pi/3); 
              sin(th)    sin(th - 2*pi/3)    sin(th + 2*pi/3) ];

v_dq = K * v_abc;

end

== matlab function bldc_sim_2024a_v1/MATLAB Function ==
  data: theta input; sector output
function sector = Sector(theta)

P = 8;
theta = mod(theta * P/2, 2*pi); % wrap around

if theta >= 0 && theta < pi/3
    sector = 1;
elseif theta >= pi/3 && theta < 2*pi/3
    sector = 2;
elseif theta >= 2*pi/3 && theta < pi
    sector = 3;
elseif theta >= pi && theta < 4*pi/3
    sector = 4;
elseif theta >= 4*pi/3 && theta < 5*pi/3
    sector = 5;
else
    sector = 6;
end

== matlab function bldc_sim_2024a_v1/MATLAB Function1 ==
  data: sector input; Va output; Vdc input; Vb output; Vc output
function [Va, Vb, Vc] = sixStepInverter(sector, Vdc)

    states = int8([ 1 -1  0;   % sector 1
                    1  0 -1;   % sector 2
                    0  1 -1;   % sector 3
                   -1  1  0;   % sector 4
                   -1  0  1;   % sector 5
                    0 -1  1]); % sector 6


    

    Va = double(states(sector,1)) * (Vdc/2);
    Vb = double(states(sector,2)) * (Vdc/2);
    Vc = double(states(sector,3)) * (Vdc/2);
end
